simulink model "lab2_simulation"  (R2025b)
settings: Solver=VariableStepAuto  StartTime=0.0  StopTime=10.0  RelTol=1e-3
settings Model: Creator=MTMTAD006  LastModifiedBy=MTMTAD006

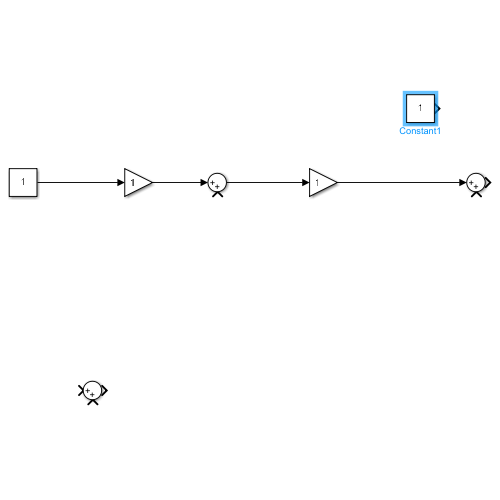
[thumbnail: Simulink's stored preview of the top-level diagram]
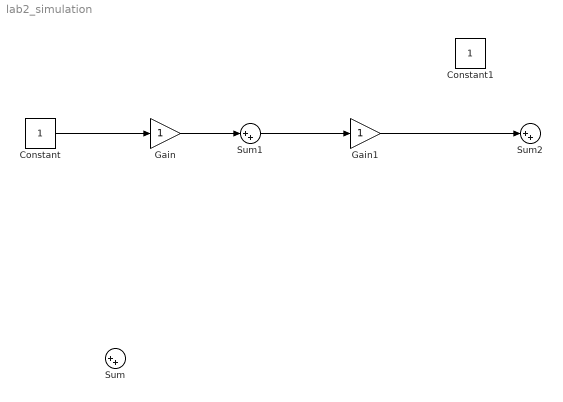
== system lab2_simulation ==
  Constant : Constant
  Constant1 : Constant
  Gain : Gain
  Gain1 : Gain
  Sum : Sum  Inputs=|++
  Sum1 : Sum  Inputs=|++
  Sum2 : Sum  Inputs=|++
  wires:
  Sum1/1 -> Gain1/1
  Gain/1 -> Sum1/1
  Constant/1 -> Gain/1
  Gain1/1 -> Sum2/1
